simulink model "LimberoGrieel_Robot_Control"  (R2022a)
settings: Solver=VariableStepAuto  StartTime=0.0  StopTime=10.0  RelTol=1e-3
values from neighbouring files (symbols this model uses):
  a = annotation('textbox',dim,'String',str,'FontSize', 20, 'FitBoxToText','on', 'Interpreter', 'tex')    [Experiment_Plot_csv.m]    (also in GRIEEL_transform.m; Gazebo_Plot_csv.m; Grasshopper_Manipulability.m = [a_1; a_2; a_3]; Hexapod_Manipulability_Develop_limits.m = [0, a2, a3])
  alpha = [alpha; alpha; alpha]    [Grasshopper_Manipulability.m]    (also in Hexapod_Manipulability_Develop_limits.m = [-pi/2, 0, 0]; LimberoGrieel_Leg_DH_Modeling_Control.m = [-pi/2,0,0,-pi/2,pi/2, -pi/2, 0]; NewLimbManipulabilityTest.m = [-pi/2, 0, 0]; NewRobot_Manipulability_Develop.m = [-pi/2, 0, 0])
  d = [d; d; d; d]    [Grasshopper_Manipulability.m]    (also in Hexapod_Manipulability_Develop_limits.m = [0, 0, 0]; LimberoGrieel_Leg_DH_Modeling_Control.m = [0,0,0,0,d5,0,d7]; NewLimbManipulabilityTest.m = [d1, 0, 0]; NewRobot_Manipulability_Develop.m = [0,0,0])
  kpp = w_cp    (= 10)    [LimberoGrieel_Leg_DH_Modeling_Control.m]    (also in limberoGrieel_leg_DH.m = 20; limbero_controller.mat; limbero_grieel_dh.m = 20)
  kpv = zeros(1,7)    [LimberoGrieel_Leg_DH_Modeling_Control.m]    (also in limberoGrieel_leg_DH.m; limbero_controller.mat = [361.812023748 321.153278445 225.192840226 266.564703352 222; limbero_grieel_dh.m)
  masses = zeros(N_link,1)    [LimberoGrieel_Leg_DH_Modeling_Control.m]    (also in limberoGrieel_leg_DH.m; limbero_controller.mat = [0.09109 0.12821 0.061841 0.081999 0.110299813858 0.13265995; limbero_grieel_dh.m)
  offset = [offset; offset; offset]    [Grasshopper_Manipulability.m]    (also in Hexapod_Manipulability_Develop_limits.m = [0, 0, 0]; LimberoGrieel_Leg_DH_Modeling_Control.m = zeros(N_link,1); NewLimbManipulabilityTest.m = [0, 0, 0]; NewRobot_Manipulability_Develop.m = [0, 0, 0])
  q0_contact = {}    [LimberoGrieel_Leg_DH_Modeling_Control.m]    (also in LimberoGrieel_Manipulability_Develop.m = q0; LimberoGrieel_Manipulability_Develop_limits.m = q0_wheel; LimberoGrieel_Manipulability_Develop_mesh.m = q0_wheel; LimberoGrieel_Manipulability_Transform.m = q0_wheel)
  r_cm = zeros(N_link,3)    [LimberoGrieel_Leg_DH_Modeling_Control.m]    (also in limberoGrieel_leg_DH.m; limbero_controller.mat = [-0.015062 -0.09917 -0.09702 -9.53000073933e-12 -0.012686054; limbero_grieel_dh.m)
  ROBOT = Robot_model(W, L, Limb, q0, [1 1 1 1], T_tool)    [Experiment_Plot_csv.m]    (also in Gazebo_Plot_csv.m; Grasshopper_Manipulability.m = Robot_model_general(W, L, Limbs, limbs_place,limbs_angle, q0; Hexapod_Manipulability_Develop_limits.m = Robot_model_general(W, L, Limbs, limbs_place,limbs_angle, q0; LimberoGrieel_Manipulability_Develop.m = Robot_model(W, L, Limb, q0_contact_swing, [1 1 1 1], T_tool))
  T_lpf = 1/(w_lpf*2*pi)    (= 0.0106103295395)    [LimberoGrieel_Leg_DH_Modeling_Control.m]    (also in limberoGrieel_leg_DH.m; limbero_controller.mat; limbero_grieel_dh.m)
  T_vel = 1/(w_vel*2*pi)    (= 0.00318309886184)    [LimberoGrieel_Leg_DH_Modeling_Control.m]    (also in limberoGrieel_leg_DH.m; limbero_controller.mat; limbero_grieel_dh.m)
  Tc = Tiv*0.1    (= 0.0666666666667)    [LimberoGrieel_Leg_DH_Modeling_Control.m]    (also in limberoGrieel_leg_DH.m = 0.0333333333333; limbero_controller.mat; limbero_grieel_dh.m = 0.0333333333333)
  Tiv = Tiv*10    (= 0.666666666667)    [LimberoGrieel_Leg_DH_Modeling_Control.m]    (also in limberoGrieel_leg_DH.m = 0.333333333333; limbero_controller.mat; limbero_grieel_dh.m = 0.333333333333)
libraries: roblocks x12
(part 2 of 2)

== system LimberoGrieel_Robot_Control/Axis Control 4/Axis7  ==
  qmd7 : Inport
  qm7 : Inport  Port=2
  tau_diff : Inport  Port=3
  wm7 : Inport  Port=4
  Add : Sum  Inputs=++-
  Add1 : Sum
  Gain : Gain  Gain=kpv(1)
  Gain1 : Gain  Gain=kpv(1)/Tiv
  Gain2 : Gain  Gain=1/Tc
  Integrator : Integrator
  Prop 7 : Gain  Gain=kpp
  Sum : Sum  Inputs=|+-
  Sum1 : Sum  Inputs=|++
  Transfer Fcn : TransferFcn  Numerator=[1 0]  Denominator=[T_vel 1]
  taum7 : Outport  VectorParamsAs1DForOutWhenUnconnected=off
  wires:
  qmd7/1 -> Transfer Fcn/1, Sum/1
  Prop 7/1 -> Add/2
  qm7/1 -> Sum/2
  Sum/1 -> Prop 7/1
  wm7/1 -> Add/3
  Transfer Fcn/1 -> Add/1
  Sum1/1 -> Integrator/1
  Gain1/1 -> Sum1/1
  Gain/1 -> Add1/1
  Add/1 -> Gain1/1, Gain/1
  tau_diff/1 -> Gain2/1
  Integrator/1 -> Add1/2
  Add1/1 -> taum7/1
  Gain2/1 -> Sum1/2

== matlab function LimberoGrieel_Robot_Control/MATLAB Function1 ==
  data: q input; g output; d parameter; a parameter; alpha parameter; offset parameter; r_cm parameter; masses parameter
function g = fcn(q, d, a, alpha, offset, r_cm, masses)
g = Gravity_compensation(a,d,alpha,offset, r_cm, masses, q, 0);

== matlab function LimberoGrieel_Robot_Control/MATLAB Function ==
  data: q input; g output; d parameter; a parameter; alpha parameter; offset parameter; r_cm parameter; masses parameter
function g = fcn(q, d, a, alpha, offset, r_cm, masses)
g = Gravity_compensation(a,d,alpha,offset, r_cm, masses, q, 0);

== matlab function LimberoGrieel_Robot_Control/MATLAB Function2 ==
  data: q input; g output; d parameter; a parameter; alpha parameter; offset parameter; r_cm parameter; masses parameter
function g = fcn(q, d, a, alpha, offset, r_cm, masses)
g = Gravity_compensation(a,d,alpha,offset, r_cm, masses, q, 0);

== matlab function LimberoGrieel_Robot_Control/MATLAB Function3 ==
  data: q input; g output; d parameter; a parameter; alpha parameter; offset parameter; r_cm parameter; masses parameter
function g = fcn(q, d, a, alpha, offset, r_cm, masses)
g = Gravity_compensation(a,d,alpha,offset, r_cm, masses, q, 0);

== matlab function LimberoGrieel_Robot_Control/check_contact ==
  data: T_limb input; contact output
function contact = fcn(T_limb)
if T_limb(4,3) <= 0 
    contact = 1; 
else 
    contact = 0; 
end

== matlab function LimberoGrieel_Robot_Control/check_contact1 ==
  data: T_limb input; contact output
function contact = fcn(T_limb)
if T_limb(4,3) <= 0 
    contact = 1; 
else 
    contact = 0; 
end

== matlab function LimberoGrieel_Robot_Control/check_contact2 ==
  data: T_limb input; contact output
function contact = fcn(T_limb)
if T_limb(4,3) <= 0 
    contact = 1; 
else 
    contact = 0; 
end

== matlab function LimberoGrieel_Robot_Control/check_contact3 ==
  data: T_limb input; contact output
function contact = fcn(T_limb)
if T_limb(4,3) <= 0 
    contact = 1; 
else 
    contact = 0; 
end
